simulink model "adc_soc_epwm_am261x"  (R2024b)
settings: Solver=FixedStepAuto  StartTime=0.0  StopTime=10.0  RelTol=1e-3
undefined symbols (not defined in the file): SYSCLOCKOUT
libraries: peripheral_library_blocks_am261x x4, HWI_lib x1
settings Model: Creator=a0499511  LastModifiedBy=a0499511
settings OptimizationCC: DefaultParameterBehavior=Inlined  EnhancedBackFolding=on  PassReuseOutputArgsAs=Individual arguments  ZeroExternalMemoryAtStartup=off  ZeroInternalMemoryAtStartup=off  MaxStackSize=64  OptimizeBlockOrder=speed  DifferentSizesBufferReuse=on  OptimizationCustomize=off  EfficientTunableParamExpr=on
settings DebuggingCC: ParameterTunabilityLossMsg=error
settings HardwareCC: ProdBitPerPointer=32  ProdBitPerSizeT=32  ProdBitPerPtrDiffT=32  ProdLargestAtomicInteger=Long  ProdLargestAtomicFloat=Double  ProdWordSize=32  ProdHWDeviceType=ARM Compatible->ARM Cortex
settings SFSimCC: MATLABDynamicMemAlloc=off
settings RTWCC: Description=Embedded Coder  SystemTargetFile=ert.tlc  HardwareBoard=AM261X LP  TemplateMakefile=ert_default_tmf  Toolchain=TI ARM Clang Compiler AM261x | gmake
settings CodeAppCC: ForceParamTrailComments=on  IgnoreCustomStorageClasses=off  OperatorAnnotations=on  SimulinkDataObjDesc=on  SFDataObjDesc=on  InsertBlockDesc=on
settings ERTTargetCC: SupportVariableSizeSignals=on  ExtModeTransport=3  ExtModeStaticAlloc=on  ExtModeMexFile=ext_xcp  ExtModeIntrfLevel=Level2 - Open  ERTCustomFileTemplate=AM263x_codertarget_file_process.tlc

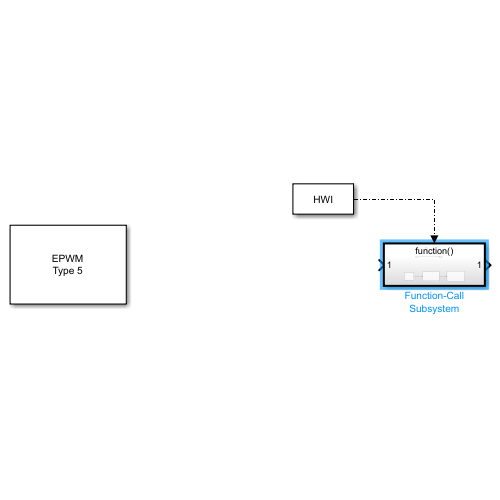
[thumbnail: Simulink's stored preview of the top-level diagram]
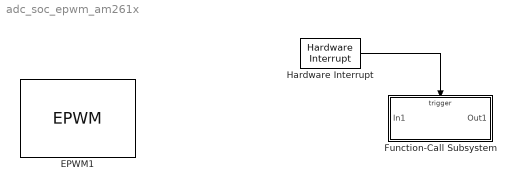
== system adc_soc_epwm_am261x ==
  EPWM1 : peripheral_library_blocks_am261x/EPWM  ePWMModule=EPWM0  ePWMLink=Disable Linking  TimerPeriodUnits=Clock Cycles  SpecifyTimerPeriod=Specify Via Dialog Box  Timer_Period=4000  Timer_Initial_Period=0  Enable_TimeBase_Global_Load_Mode=off  PeriodLoadMode=Using Shadow registers  PeriodLoadEvent=Shadow to Active load when counter reaches zero  EmulationMode=Stop after next Time Base Counter increaments or decreaments  TBCLK=Divide clock by 4  HSPCLKDIV=Divide clock by 8  CounterMode=Up count  CounterInitialValue=0  Phase_Shift_Load_Enable=off  Phase_Shift_Value=0  SyncInPulseSrc=Disable Sync-in  Software_Force_EPWM_SyncOut_Pulse=off  Counter_Zero_EPWM_SyncOut_Pulse=off  Counter_CMPB_EPWM_SyncOut_Pulse=off  Counter_CMPC_EPWM_SyncOut_Pulse=off  Counter_CMPD_EPWM_SyncOut_Pulse=off  DCA_Event1_Sync_Signal=off  DCB_Event1_Sync_Signal=off  OneShotTrigger=Trigger is one-shot sync  Enable_LinkCounterCMPA=off  ePWMLinkCMPA=Link with ePWM0  CMPAUnits=Clock Cycles  SpecifyCMPAVia=Specify Via Dialog Box  CMPAValue=1000  CMPA_Initial_Value=0  Enable_Global_Load_CMPA=off  Enable_Shadow_Load_CMPA=on  SHDWAMODE=Load when counter equals zero  Enable_LinkCounterCMPB=off  ePWMLinkCMPB=Link with ePWM0  CMPBUnits=Clock Cycles  SpecifyCMPBVia=Specify Via Dialog Box  CMPBValue=0  CMPB_Initial_Value=0  Enable_Global_Load_CMPB=off  Enable_Shadow_Load_CMPB=on  SHDWBMODE=Load when counter equals zero  Enable_LinkCounterCMPC=off  ePWMLinkCMPC=Link with ePWM0  CMPCUnits=Clock Cycles  SpecifyCMPCVia=Specify Via Dialog Box  CMPCValue=0  CMPC_Initial_Value=0  Enable_Global_Load_CMPC=off  Enable_Shadow_Load_CMPC=on  SHDWCMODE=Load when counter equals zero  Enable_LinkCounterCMPD=off  ePWMLinkCMPD=Link with ePWM0  CMPDUnits=Clock Cycles  SpecifyCMPDVia=Specify Via Dialog Box  CMPDValue=0  CMPD_Initial_Value=0  Enable_Global_Load_CMPD=off  Enable_Shadow_Load_CMPD=on  SHDWDMODE=Load when counter equals zero  Enable_Software_Force_Global_Load=off  SoftwareForceShadowMode=Shadow mode load when counter equals zero  T1TriggerSource=Digital compare event A 1  T2TriggerSource=Digital compare event A 1  EnableePWMXAGlobalLoad=off  Enable_ePWMXA_Shadow_Mode=off  ePWMXAShadowLoadEvent=Load when counter equals zero  ePWMXAOneTimeSWForceAction=No change in output pins  ePWMXAContinuousSWForceAction=Software forcing disabled  ePWMXATbctrZero=No change in output pins  ePWMXATbctrPrd=No change in output pins  ePWMXATbctrCMPAUp=No change in output pins  ePWMXATbctrCMPADown=No change in output pins  ePWMXATbctrCMPBUp=No change in output pins  ePWMXATbctrCMPBDown=No change in output pins  ePWMXAT1Up=No change in output pins  ePWMXAT1Down=No change in output pins  ePWMXAT2Up=No change in output pins  ePWMXAT2Down=No change in output pins  EnableePWMXBGlobalLoad=off  Enable_ePWMXB_Shadow_Mode=off  ePWMXBShadowLoadEvent=Load when counter equals zero  ePWMXBOneTimeSWForceAction=No change in output pins  ePWMXBContinuousSWForceAction=Software forcing disabled  ePWMXBTbctrZero=No change in output pins  ePWMXBTbctrPrd=No change in output pins  ePWMXBTbctrCMPAUp=No change in output pins  ePWMXBTbctrCMPADown=No change in output pins  ePWMXBTbctrCMPBUp=No change in output pins  ePWMXBTbctrCMPBDown=No change in output pins  ePWMXBT1Up=No change in output pins  ePWMXBT1Down=No change in output pins  ePWMXBT2Up=No change in output pins  ePWMXBT2Down=No change in output pins  Use_Advanced_EPWM_Trip_Zone_Actions=off  TZAEvent=High impedance output  TZBEvent=High impedance output  DCAEVT1Event=High impedance output  DCAEVT2Event=High impedance output  DCBEVT1Event=High impedance output  DCBEVT2Event=High impedance output  TZBDEvent=High impedance output  TZBUEvent=High impedance output  TZADEvent=High impedance output  TZAUEvent=High impedance output  DCAEVT1UEvent=High impedance output  DCAEVT1DEvent=High impedance output  DCAEVT2UEvent=High impedance output  DCAEVT2DEvent=High impedance output  DCBEVT1UEvent=High impedance output  DCBEVT1DEvent=High impedance output  DCBEVT2UEvent=High impedance output  DCBEVT2DEvent=High impedance output  One_Shot_TZ1=off  One_Shot_TZ2=off  One_Shot_TZ3=off  One_Shot_TZ4=off  One_Shot_TZ5=off  One_Shot_TZ6=off  One_Shot_DCAEVT1=off  One_Shot_DCBEVT1=off  TZ1_Cycle_By_Cycle=off  TZ2_Cycle_By_Cycle=off  TZ3_Cycle_By_Cycle=off  TZ4_Cycle_By_Cycle=off  TZ5_Cycle_By_Cycle=off  TZ6_Cycle_By_Cycle=off  DCAEVT2_Cycle_By_Cycle=off  DCBEVT2_Cycle_By_Cycle=off  CBCLatchClearSignal=Clear CBC Pulse when counter reaches zero  Trip_Zones_Cycle_By_Cycle_interrupt=off  Trip_Zones_One_Shot_interrupt=off  Digital_CompareA_Event1_interrupt=off  Digital_CompareA_Event2_interrupt=off  Digital_CompareB_Event1_interrupt=off  Digital_CompareB_Event2_interrupt=off  DCAHigh=Trip 1  DCAHigh_CombTrip1_Input=off  DCAHigh_CombTrip2_Input=off  DCAHigh_CombTrip3_Input=off  DCAHigh_CombTrip4_Input=off  DCAHigh_CombTrip5_Input=off  DCAHigh_CombTrip6_Input=off  DCAHigh_CombTrip7_Input=off  DCAHigh_CombTrip8_Input=off  DCAHigh_CombTrip9_Input=off  DCAHigh_CombTrip10_Input=off  DCAHigh_CombTrip11_Input=off  DCAHigh_CombTrip12_Input=off  DCAHigh_CombTrip13_Input=off  DCAHigh_CombTrip14_Input=off  DCAHigh_CombTrip15_Input=off  DCALow=Trip 1  DCALow_CombTrip1_Input=off  DCALow_CombTrip2_Input=off  DCALow_CombTrip3_Input=off  DCALow_CombTrip4_Input=off  DCALow_CombTrip5_Input=off  DCALow_CombTrip6_Input=off  DCALow_CombTrip7_Input=off  DCALow_CombTrip8_Input=off  DCALow_CombTrip9_Input=off  DCALow_CombTrip10_Input=off  DCALow_CombTrip11_Input=off  DCALow_CombTrip12_Input=off  DCALow_CombTrip13_Input=off  DCALow_CombTrip14_Input=off  DCALow_CombTrip15_Input=off  DCOutput1ACondition=Event is disabled  DCOutput2ACondition=Event is disabled  SynchModeDCAEVT1=DC Input signal is synced with TBCLK  SignalSourceDCAEVT1=Signal source is unfiltered  CBCLatchModeDCAEVT1=DC CBC latch is disabled  CBCLatchClearEventDCAEVT1=Clear CBC latch when counter equals zero  SynchModeDCAEVT2=DC Input signal is synced with TBCLK  SignalSourceDCAEVT2=Signal source is unfiltered  CBCLatchModeDCAEVT2=DC CBC latch is disabled  CBCLatchClearEventDCAEVT2=Clear CBC latch when counter equals zero  DCBHigh=Trip 1  DCBHigh_CombTrip1_Input=off  DCBHigh_CombTrip2_Input=off  DCBHigh_CombTrip3_Input=off  DCBHigh_CombTrip4_Input=off  DCBHigh_CombTrip5_Input=off  DCBHigh_CombTrip6_Input=off  DCBHigh_CombTrip7_Input=off  DCBHigh_CombTrip8_Input=off  DCBHigh_CombTrip9_Input=off  DCBHigh_CombTrip10_Input=off  DCBHigh_CombTrip11_Input=off  DCBHigh_CombTrip12_Input=off  DCBHigh_CombTrip13_Input=off  DCBHigh_CombTrip14_Input=off  DCBHigh_CombTrip15_Input=off  DCBLow=Trip 1  DCBLow_CombTrip1_Input=off  DCBLow_CombTrip2_Input=off  DCBLow_CombTrip3_Input=off  DCBLow_CombTrip4_Input=off  DCBLow_CombTrip5_Input=off  DCBLow_CombTrip6_Input=off  DCBLow_CombTrip7_Input=off  DCBLow_CombTrip8_Input=off  DCBLow_CombTrip9_Input=off  DCBLow_CombTrip10_Input=off  DCBLow_CombTrip11_Input=off  DCBLow_CombTrip12_Input=off  DCBLow_CombTrip13_Input=off  DCBLow_CombTrip14_Input=off  DCBLow_CombTrip15_Input=off  DCOutput1BCondition=Event is disabled  DCOutput2BCondition=Event is disabled  SynchModeDCBEVT1=DC Input signal is synced with TBCLK  SignalSourceDCBEVT1=Signal source is unfiltered  CBCLatchModeDCBEVT1=DC CBC latch is disabled  CBCLatchClearEventDCBEVT1=Clear CBC latch when counter equals zero  SynchModeDCBEVT2=DC Input signal is synced with TBCLK  SignalSourceDCBEVT2=Signal source is unfiltered  CBCLatchModeDCBEVT2=DC CBC latch is disabled  CBCLatchClearEventDCBEVT2=Clear CBC latch when counter equals zero  DCFilterInputEventSource=DC filter signal source is DCAEVT1  Blanking_Window_Usage=off  BlankingWindowStartEvent=Time base counter equals period  BlankingWindow_MixedEvent_TBCTRZero=off  BlankingWindow_MixedEvent_TBCTRPrd=off  BlankingWindow_MixedEvent_TBCTRCMPA_Inc=off  BlankingWindow_MixedEvent_TBCTRCMPA_Dec=off  BlankingWindow_MixedEvent_TBCTRCMPB_Inc=off  BlankingWindow_MixedEvent_TBCTRCMPB_Dec=off  BlankingWindow_MixedEvent_TBCTRCMPC_Inc=off  BlankingWindow_MixedEvent_TBCTRCMPC_Dec=off  BlankingWindow_MixedEvent_TBCTRCMPD_Inc=off  BlankingWindow_MixedEvent_TBCTRCMPD_Dec=off  Blanking_Window_Offset=0  Blanking_Window_Length=0  Invert_Blanking_Window=off  Enable_DC_Counter_Capture=off  Enable_Counter_Capture_Shadow_Mode=off  DCCounterCaptureEnableEvent=Time base counter equals period  Use_Edge_Filter=off  EdgeFilterMode=Digital Compare Edge Filter low  EdgeFilterEdgeCount=No edge is required to generate event  Enable_Edge_Filter_Valley_Capture=off  EdgeFilterCounterCaptureSignal=Valley capture triggered by software  Start_Valley_Capture_Logic=off  StartValleyCapture=0 Event  StopValleyCapture=0 Event  Select_Delayed_Output_of_Edge_Filter=off  Software_Valley_Delay_Value=0  ValleyDelayDivider=Delay value equals offset value defined by software  Use_Event_Detection=off  Capture_Input=Trip 1  Invert_Capture_Input_Polarity=Capture input is not inverted  Capture_gate=Trip 1  Capture_gate_polarity_select=Capture gate is always on  Combinational_capture_input_Trip1=off  Combinational_capture_input_Trip2=off  Combinational_capture_input_Trip3=off  Combinational_capture_input_Trip4=off  Combinational_capture_input_Trip5=off  Combinational_capture_input_Trip6=off  Combinational_capture_input_Trip7=off  Combinational_capture_input_Trip8=off  Combinational_capture_input_Trip9=off  Combinational_capture_input_Trip10=off  Combinational_capture_input_Trip11=off  Combinational_capture_input_Trip12=off  Combinational_capture_input_Trip13=off  Combinational_capture_input_Trip14=off  Combinational_capture_input_Trip15=off  Combinational_capture_gate_Trip1=off  Combinational_capture_gate_Trip2=off  Combinational_capture_gate_Trip3=off  Combinational_capture_gate_Trip4=off  Combinational_capture_gate_Trip5=off  Combinational_capture_gate_Trip6=off  Combinational_capture_gate_Trip7=off  Combinational_capture_gate_Trip8=off  Combinational_capture_gate_Trip9=off  Combinational_capture_gate_Trip10=off  Combinational_capture_gate_Trip11=off  Combinational_capture_gate_Trip12=off  Combinational_capture_gate_Trip13=off  Combinational_capture_gate_Trip14=off  Combinational_capture_gate_Trip15=off  RisingEdgeDelayInput=Input signal is ePWMA  FallingEdgeDelayInput=Input signal is ePWMA  RisingEdgeDelayPolarity=DB polarity is not inverted  FallingEdgeDelayPolarity=DB polarity is not inverted  DeadBandCounterClockRate=Deadband counter runs at TBCLK rate  Enable_Rising_Edge_Delay=off  Rising_Edge_Delay_Value=0  Enable_Falling_Edge_Delay=off  Falling_Edge_Delay_Value=0  Swap_Output_for_EPWMxA=off  Swap_Output_for_EPWMxB=off  EnableDeadbandControlShadowMode=off  DeadbandControlShadowMode=Load when counter equals zero  Enable_Deadband_Control_Global_Load=off  Enable_RED_Shadow_Mode=off  REDShadowLoadEvent=Load when counter equals zero  Enable_RED_Global_Load=off  Enable_FED_Shadow_Mode=off  FEDShadowLoadEvent=Load when counter equals zero  Enable_FED_Global_Load=off  Use_Chopper=off  ChopperDutyCycle=1/8 Duty  ChopperFrequency=SYSCLOCKOUT/1  ChopperFirstPulseWidth=1  Enable_EPWM_Interrupt=off  InterruptEventSources=Time base counter equal to zero  EventTrigger_MixedEvent_TBCTRZero=off  EventTrigger_MixedEvent_TBCTRPrd=off  EventTrigger_MixedEvent_TBCTRCMPA_Inc=off  EventTrigger_MixedEvent_TBCTRCMPA_Dec=off  EventTrigger_MixedEvent_TBCTRCMPB_Inc=off  EventTrigger_MixedEvent_TBCTRCMPB_Dec=off  EventTrigger_MixedEvent_TBCTRCMPC_Inc=off  EventTrigger_MixedEvent_TBCTRCMPC_Dec=off  EventTrigger_MixedEvent_TBCTRCMPD_Inc=off  EventTrigger_MixedEvent_TBCTRCMPD_Dec=off  EventTrigger_MixedEvent_DCxEVT1=off  InterruptEventCount=Disabled  Enable_Interrupt_Event_Count_Initial_Value=off  InterruptEventCountInitialValue=Initialize event counter to 0  SOCA_Trigger_Enable=on  SOCATriggerSource=Time base counter equal to CMPA when timer is incrementing  SOCATrigger_MixedEvent_TBCTRZero=off  SOCATrigger_MixedEvent_TBCTRPrd=off  SOCATrigger_MixedEvent_TBCTRCMPA_Inc=off  SOCATrigger_MixedEvent_TBCTRCMPA_Dec=off  SOCATrigger_MixedEvent_TBCTRCMPB_Inc=off  SOCATrigger_MixedEvent_TBCTRCMPB_Dec=off  SOCATrigger_MixedEvent_TBCTRCMPC_Inc=off  SOCATrigger_MixedEvent_TBCTRCMPC_Dec=off  SOCATrigger_MixedEvent_TBCTRCMPD_Inc=off  SOCATrigger_MixedEvent_TBCTRCMPD_Dec=off  SOCATrigger_MixedEvent_DCxEVT1=off  SOCATriggerEventCount=1 event generates interrupt  SOCA_Trigger_Event_Count_Init_Enable=off  SOCATriggerEventCountInitValue=Initialize event counter to 0  SOCB_Trigger_Enable=off  SOCBTriggerSource=Event is based on DCxEVT1  SOCBTrigger_MixedEvent_TBCTRZero=off  SOCBTrigger_MixedEvent_TBCTRPrd=off  SOCBTrigger_MixedEvent_TBCTRCMPA_Inc=off  SOCBTrigger_MixedEvent_TBCTRCMPA_Dec=off  SOCBTrigger_MixedEvent_TBCTRCMPB_Inc=off  SOCBTrigger_MixedEvent_TBCTRCMPB_Dec=off  SOCBTrigger_MixedEvent_TBCTRCMPC_Inc=off  SOCBTrigger_MixedEvent_TBCTRCMPC_Dec=off  SOCBTrigger_MixedEvent_TBCTRCMPD_Inc=off  SOCBTrigger_MixedEvent_TBCTRCMPD_Dec=off  SOCBTrigger_MixedEvent_DCxEVT1=off  SOCBTriggerEventCount=Disabled  SOCB_Trigger_Event_Count_Init_Enable=off  SOCBTriggerEventCountInitValue=Initialize event counter to 0  Enable_HRPWM_Support=off  Enable_Automatic_HRMSTEP_Scaling=off  Enable_SFO=off  MEP_Scale=0  ControlModeChannelA=CMPAHR/CMPBHR or TBPRDHR controls MEP edge  ControlModeChannelB=CMPAHR/CMPBHR or TBPRDHR controls MEP edge  HRPWM_High_Resolution_Phase=0  High_Resolution_Phase_Load_Enable=off  HRPWMChannelAEdgeMode=HRPWM is disabled  High_Resolution_CMPA=1  CMPAHRShadowToActiveLoadEvent=Load when counter equals zero  HRPWMChannelBEdgeMode=HRPWM is disabled  High_Resolution_CMPB=1  CMPBHRShadowToActiveLoadEvent=Load when counter equals zero  HRPWM_High_Resolution_Period_Enable=off  HRPWM_High_Resolution_Period=0  HRPWMDeadbandEdgeMode=HRPWM is disabled  HRPWM_High_Resolution_RED=0  ShadowActiveLoadDBREDHR=Load when counter equals zero  HRPWM_High_Resolution_FED=0  ShadowActiveLoadDBFEDHR=Load when counter equals zero  Swap_A_B_Outputs=off  EPWMxBOutputSelect=ePWMxB output is normal  Enable_XCMP_Mode=off  Enable_Split_XCMP=off  Allocate_XCMP_CMPA=Allocate 0 XCMP registers to CMPA  Allocate_XCMP_CMPB=Allocate XCMP5 register to CMPB  SpecifyXCMPActive=Specify via Dialog Box  XCMP1_Active=0  XCMP2_Active=0  XCMP3_Active=0  XCMP4_Active=0  XCMP5_Active=0  XCMP6_Active=0  XCMP7_Active=0  XCMP8_Active=0  XCMP1_Active_Initial=0  XCMP2_Active_Initial=0  XCMP3_Active_Initial=0  XCMP4_Active_Initial=0  XCMP5_Active_Initial=0  XCMP6_Active_Initial=0  XCMP7_Active_Initial=0  XCMP8_Active_Initial=0  SpecifyXCMPShadow1=Specify via Dialog Box  XCMP1_SHADOW1=0  XCMP2_SHADOW1=0  XCMP3_SHADOW1=0  XCMP4_SHADOW1=0  XCMP5_SHADOW1=0  XCMP6_SHADOW1=0  XCMP7_SHADOW1=0  XCMP8_SHADOW1=0  XCMP1_SHADOW1_Initial=0  XCMP2_SHADOW1_Initial=0  XCMP3_SHADOW1_Initial=0  XCMP4_SHADOW1_Initial=0  XCMP5_SHADOW1_Initial=0  XCMP6_SHADOW1_Initial=0  XCMP7_SHADOW1_Initial=0  XCMP8_SHADOW1_Initial=0  SpecifyXCMPShadow2=Specify via Dialog Box  XCMP1_SHADOW2=0  XCMP2_SHADOW2=0  XCMP3_SHADOW2=0  XCMP4_SHADOW2=0  XCMP5_SHADOW2=0  XCMP6_SHADOW2=0  XCMP7_SHADOW2=0  XCMP8_SHADOW2=0  XCMP1_SHADOW2_Initial=0  XCMP2_SHADOW2_Initial=0  XCMP3_SHADOW2_Initial=0  XCMP4_SHADOW2_Initial=0  XCMP5_SHADOW2_Initial=0  XCMP6_SHADOW2_Initial=0  XCMP7_SHADOW2_Initial=0  XCMP8_SHADOW2_Initial=0  SpecifyXCMPShadow3=Specify via Dialog Box  XCMP1_SHADOW3=0  XCMP2_SHADOW3=0  XCMP3_SHADOW3=0  XCMP4_SHADOW3=0  XCMP5_SHADOW3=0  XCMP6_SHADOW3=0  XCMP7_SHADOW3=0  XCMP8_SHADOW3=0  XCMP1_SHADOW3_Initial=0  XCMP2_SHADOW3_Initial=0  XCMP3_SHADOW3_Initial=0  XCMP4_SHADOW3_Initial=0  XCMP5_SHADOW3_Initial=0  XCMP6_SHADOW3_Initial=0  XCMP7_SHADOW3_Initial=0  XCMP8_SHADOW3_Initial=0  EPWMXA_tbctr_XCMP1_active=No change in output pins  EPWMXA_tbctr_XCMP2_active=No change in output pins  EPWMXA_tbctr_XCMP3_active=No change in output pins  EPWMXA_tbctr_XCMP4_active=No change in output pins  EPWMXA_tbctr_XCMP5_active=No change in output pins  EPWMXA_tbctr_XCMP6_active=No change in output pins  EPWMXA_tbctr_XCMP7_active=No change in output pins  EPWMXA_tbctr_XCMP8_active=No change in output pins  EPWMXB_tbctr_XCMP5_active=No change in output pins  EPWMXB_tbctr_XCMP6_active=No change in output pins  EPWMXB_tbctr_XCMP7_active=No change in output pins  EPWMXB_tbctr_XCMP8_active=No change in output pins  EPWMXA_tbctr_XCMP1_SHADOW1=No change in output pins  EPWMXA_tbctr_XCMP2_SHADOW1=No change in output pins  EPWMXA_tbctr_XCMP3_SHADOW1=No change in output pins  EPWMXA_tbctr_XCMP4_SHADOW1=No change in output pins  EPWMXA_tbctr_XCMP5_SHADOW1=No change in output pins  EPWMXA_tbctr_XCMP6_SHADOW1=No change in output pins  EPWMXA_tbctr_XCMP7_SHADOW1=No change in output pins  EPWMXA_tbctr_XCMP8_SHADOW1=No change in output pins  EPWMXB_tbctr_XCMP5_SHADOW1=No change in output pins  EPWMXB_tbctr_XCMP6_SHADOW1=No change in output pins  EPWMXB_tbctr_XCMP7_SHADOW1=No change in output pins  EPWMXB_tbctr_XCMP8_SHADOW1=No change in output pins  EPWMXA_tbctr_XCMP1_SHADOW2=No change in output pins  EPWMXA_tbctr_XCMP2_SHADOW2=No change in output pins  EPWMXA_tbctr_XCMP3_SHADOW2=No change in output pins  EPWMXA_tbctr_XCMP4_SHADOW2=No change in output pins  EPWMXA_tbctr_XCMP5_SHADOW2=No change in output pins  EPWMXA_tbctr_XCMP6_SHADOW2=No change in output pins  EPWMXA_tbctr_XCMP7_SHADOW2=No change in output pins  EPWMXA_tbctr_XCMP8_SHADOW2=No change in output pins  EPWMXB_tbctr_XCMP5_SHADOW2=No change in output pins  EPWMXB_tbctr_XCMP6_SHADOW2=No change in output pins  EPWMXB_tbctr_XCMP7_SHADOW2=No change in output pins  EPWMXB_tbctr_XCMP8_SHADOW2=No change in output pins  EPWMXA_tbctr_XCMP1_SHADOW3=No change in output pins  EPWMXA_tbctr_XCMP2_SHADOW3=No change in output pins  EPWMXA_tbctr_XCMP3_SHADOW3=No change in output pins  EPWMXA_tbctr_XCMP4_SHADOW3=No change in output pins  EPWMXA_tbctr_XCMP5_SHADOW3=No change in output pins  EPWMXA_tbctr_XCMP6_SHADOW3=No change in output pins  EPWMXA_tbctr_XCMP7_SHADOW3=No change in output pins  EPWMXA_tbctr_XCMP8_SHADOW3=No change in output pins  EPWMXB_tbctr_XCMP5_SHADOW3=No change in output pins  EPWMXB_tbctr_XCMP6_SHADOW3=No change in output pins  EPWMXB_tbctr_XCMP7_SHADOW3=No change in output pins  EPWMXB_tbctr_XCMP8_SHADOW3=No change in output pins  XMIN_Active=0  XMAX_Active=0  XMIN_Shadow1=0  XMAX_Shadow1=0  XMIN_Shadow2=0  XMAX_Shadow2=0  XMIN_Shadow3=0  XMAX_Shadow3=0  XTBPRD_Active=0  XTBPRD_Shadow1=0  XTBPRD_Shadow2=0  XTBPRD_Shadow3=0  Load_Mode=Load Once  Shadow_Level=Shadow level zero  Shadow_register_load_once=Do not load any shadow register set  Repeat_Count_Shadow_Buffer2=0  Repeat_Count_Shadow_Buffer3=0
  Function-Call Subsystem : Subsystem  TreatAsAtomicUnit=on
  Hardware Interrupt : HWI_lib/Hardware Interrupt  INTERRUPT_TYPE=ADC  ISR_NUMBER=168  INSTANCE_NUMBER=1  SHOW_INPUTPORT=off
      settings: SourceProductName=Embedded Coder Support Package for AM263x - HWI Block
  wires:
  Hardware Interrupt/1 -> Function-Call Subsystem/Trigger

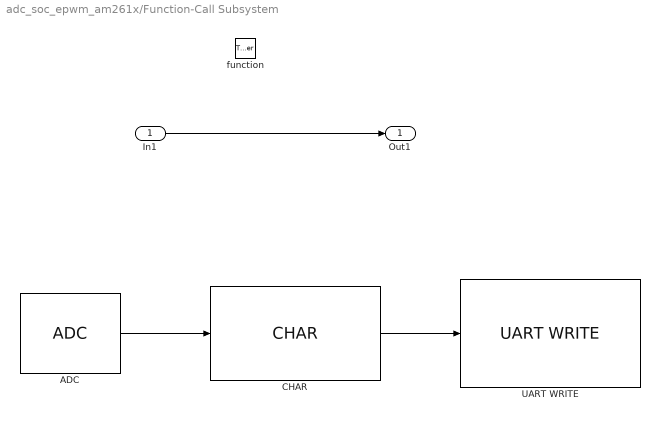
== system adc_soc_epwm_am261x/Function-Call Subsystem ==
  In1 : Inport
  function : TriggerPort  TriggerType=function-call  VariantControl=(inherit)
  ADC : peripheral_library_blocks_am261x/ADC  ADCModule=ADC1  Prescaler=3.0  ResolutionMode=Twelve bit conversion  SOCPriority=All Round Robin  SignalMode=Sample on single pin with VREFLO  SOCTriggerNo=SOC0  SOCx_acquisition_Window=20  SOCxTriggerSource=EPWM0 SOCA  INTWillTriggerSOCx=No ADCINT Trigger  DataType=Unsigned INT16  ADCEnableConverter=on  PulseMode=Pulse generation at End of Acquisition Window  PostInterruptAtEOCTrigger=on  InterruptSelection=ADC Interrupt Number 1  InterruptSOCSource=SOC0  ADCINT1CONTINOUSMODE=off  ADCINT2CONTINOUSMODE=off  ADCINT3CONTINOUSMODE=off  ADCINT4CONTINOUSMODE=off  SampleTime=-1  Channels=Channel 0  Channels1=Channels 0 and 1  PPBBlock=PPB Block 1  PPBSocEocNO=SOC0  Enable_Event_ADC_Trip_High=off  Enable_Event_ADC_Trip_Low=off  Enable_Event_ADC_Zero_Crossing=off  Enable_Interrupt_Event_ADC_Trip_High=off  Enable_Interrupt_Event_ADC_Trip_Low=off  Enable_Interrupt_Event_ADC_Zero_Crossing=off  PPBEnableTwoComplement=off  PPBEnablePPBEventCBCClear=off  PPB_Calibration_Offset=0  PPB_Reference_Offset=0  PPB_High_Trip_Limit=0  PPB_Low_Trip_Limit=0  BurstModeTrigger=Software Source  BurstSize=1 SOC long  ADCEnableBurstMode=off
  CHAR : peripheral_library_blocks_am261x/CHAR
  UART WRITE : peripheral_library_blocks_am261x/UART WRITE  UARTPort=UART0
  Out1 : Outport
  wires:
  In1/1 -> Out1/1
  ADC/1 -> CHAR/1
  CHAR/1 -> UART WRITE/1
